simulink model "sampleModel1487"  (R2023a)
settings: Solver=VariableStepAuto  StartTime=0.0  StopTime=10.0  RelTol=1e-3
libraries: hdlsllib x4, simulink x2
settings Model: Creator=user1  LastModifiedBy=user1

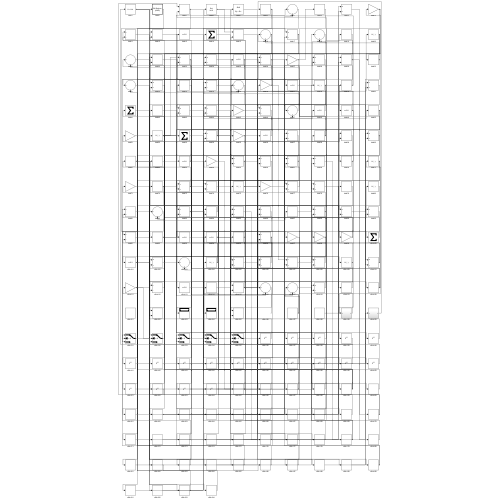
[thumbnail: Simulink's stored preview of the top-level diagram]
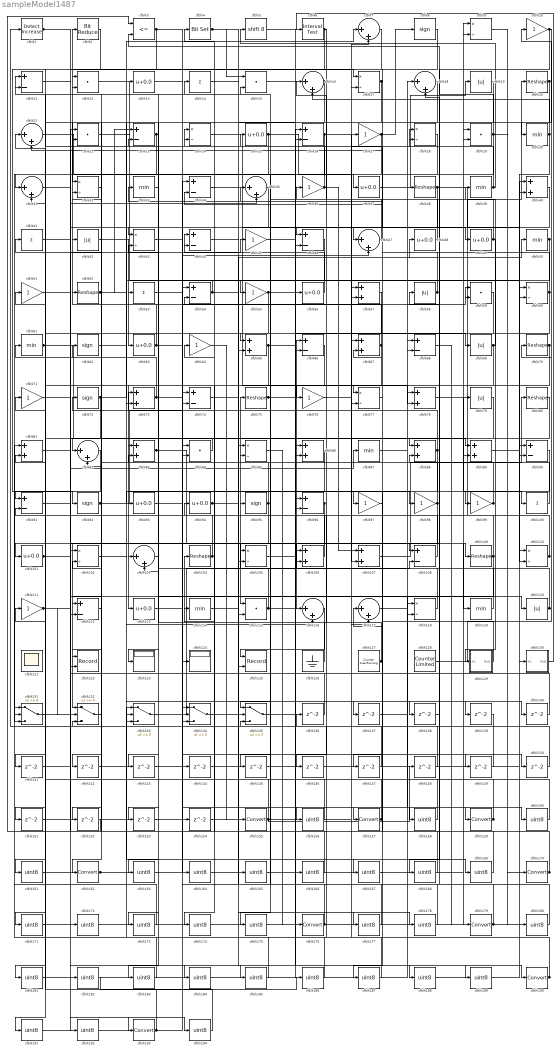
== system sampleModel1487 ==
  cfblk1 : simulink/Logic and Bit Operations/Detect Increase  vinit=0.0  OutDataTypeStr=boolean
      settings: LibrarySourceBlock=|
      | hdlsllib/Logic and Bit
      | Operations/Detect
      | Increase
  cfblk{10,27,36,45,51,55,64,71,76,97..99,111} (13 alike) : Gain
  cfblk{14,41,53,100} (4 alike) : Sum  Inputs=+
  cfblk{13,25,37,48..49,56,63,93..94,101,113} (11 alike) : Bias  Bias=0.0  SaturateOnIntegerOverflow=off
  cfblk{9,17,24,28,32,43,60,77,85,102,105,110,118} (13 alike) : Product  Inputs=*/  RndMeth=Zero  SaturateOnIntegerOverflow=on
  cfblk{7,16,18,21,31,35,47,82,103,116..117} (11 alike) : Sum  Inputs=|++
  cfblk{20,38,52,70,75,80,104,109} (8 alike) : Reshape
  cfblk{40,57,65,67,73,78,81,83,86,88..89,106..107} (13 alike) : Sum
  cfblk{11,23,26,34,44,46,54,66,68,74,90..91,96,108,112} (15 alike) : Sum  Inputs=+-
  cfblk{30,33,39,50,61,87,114,119} (8 alike) : MinMax
  cfblk{12,15,22,29,59,84,115} (7 alike) : DotProduct  OutDataTypeStr=Inherit: Inherit via internal rule
  cfblk{19,42,58,69,79,120} (6 alike) : Abs  SaturateOnIntegerOverflow=off
  cfblk121 : Scope
      settings: Floating=on
  cfblk122 : Record  FileSettingsInternal="{\"entries\":[{\"content\":{\"excelSettings\":{\"content\":{},\"type\":\"Streamout.ExcelSettings\"}},\"type\":\"Streamout.FileSettingStorage\",\"uuid\":\"\"}],\"packageUris\":[\"http:\\/\\/schema.mathworks.com\\/mf0\\/streamout_blocks\\/R2020a\"],\"version\":\"1.0\"}"  Layout=[1 1]  SignalsInternal="{\"entries\":[{\"content\":{\"signals\":[{\"content\":{\"blockPath\":[],\"dimensions\":[1],\"domain\":\"\",\"lineColor\":\"#a2142f\",\"plots\":[1],\"port\":1,\"signalID\":1175,\"signalName\":\"XY Graph:1\"},\"type\":\"RecordBlkView.Signal\",\"uuid\":\"\"},{\"content\":{\"blockPath\":[],\"dimensions\":[1],\"domain\":\"\",\"lineColor\":\"#139fff\",\"plots\":[1],\"port\":2,\"signalID\":1178,\"signalName\":\"XY Graph:2\"},\"type\":\"RecordBlkView.Signal\",\"uuid\":\"\"}]},\"type\":\"RecordBlkView.InputSignals\",\"uuid\":\"\"}],\"packageUris\":[\"http:\\/\\/schema.mathworks.com\\/mf0\\/streamout_blocks\\/R2020a\"],\"version\":\"1.0\"}"  VisualizationBindings="{\"xyplotplugin\":{\"info\":[{\"series\":[{\"bindingParametersList\":[{\"parameter\":\"X-Axis\",\"signalID\":1175,\"signalName\":\"XY Graph:1\"},{\"parameter\":\"Y-Axis\",\"signalID\":1178,\"signalName\":\"XY Graph:2\"}],\"seriesID\":46251}],\"subplotID\":1}]}}"  CompatibilityTag=XY  st=-1
  cfblk123 : Display
  cfblk124 : Display
  cfblk125 : Record  FileSettingsInternal="{\"entries\":[{\"content\":{\"excelSettings\":{\"content\":{},\"type\":\"Streamout.ExcelSettings\"}},\"type\":\"Streamout.FileSettingStorage\",\"uuid\":\"\"}],\"packageUris\":[\"http:\\/\\/schema.mathworks.com\\/mf0\\/streamout_blocks\\/R2020a\"],\"version\":\"1.0\"}"  Layout=[1 1]  SignalsInternal="{\"entries\":[{\"content\":{\"signals\":[{\"content\":{\"blockPath\":[],\"dimensions\":[1],\"domain\":\"\",\"lineColor\":\"#a2142f\",\"plots\":[1],\"port\":1,\"signalID\":1183,\"signalName\":\"XY Graph:1\"},\"type\":\"RecordBlkView.Signal\",\"uuid\":\"\"},{\"content\":{\"blockPath\":[],\"dimensions\":[1],\"domain\":\"\",\"lineColor\":\"#139fff\",\"plots\":[1],\"port\":2,\"signalID\":1186,\"signalName\":\"XY Graph:2\"},\"type\":\"RecordBlkView.Signal\",\"uuid\":\"\"}]},\"type\":\"RecordBlkView.InputSignals\",\"uuid\":\"\"}],\"packageUris\":[\"http:\\/\\/schema.mathworks.com\\/mf0\\/streamout_blocks\\/R2020a\"],\"version\":\"1.0\"}"  VisualizationBindings="{\"xyplotplugin\":{\"info\":[{\"series\":[{\"bindingParametersList\":[{\"parameter\":\"X-Axis\",\"signalID\":1183,\"signalName\":\"XY Graph:1\"},{\"parameter\":\"Y-Axis\",\"signalID\":1186,\"signalName\":\"XY Graph:2\"}],\"seriesID\":58959}],\"subplotID\":1}]}}"  CompatibilityTag=XY  st=-1
  cfblk126 : Ground
  cfblk127 : hdlsllib/Sources/Counter Free-Running  NumBits=16  tsamp=-1
  cfblk128 : hdlsllib/Sources/Counter Limited  uplimit=7  tsamp=-1
  cfblk129 : Subsystem
      settings: LibrarySourceBlock=|
      | hdlsllib/Ports &
      | Subsystems/Subsystem
  cfblk130 : Subsystem
      settings: LibrarySourceBlock=|
      | hdlsllib/Ports &
      | Subsystems/Subsystem
  cfblk{131..135} (5 alike) : Switch  SaturateOnIntegerOverflow=off  InputSameDT=off
  cfblk{136..154} (19 alike) : Delay  SampleTime=1
  cfblk{155,157,159,162,170,176,179,190,193} (9 alike) : DataTypeConversion  SaturateOnIntegerOverflow=off  RndMeth=Floor
  cfblk{156,158,160..161,163..169,171..175,177..178,180..189,191..192,194} (31 alike) : DataTypeConversion  OutDataTypeStr=uint8  SaturateOnIntegerOverflow=off  RndMeth=Floor
  cfblk2 : hdlsllib/Logic and Bit Operations/Bit Reduce  mode=AND
  cfblk3 : RelationalOperator  Operator=<=  OutDataTypeStr=boolean  InputSameDT=off
  cfblk4 : simulink/Logic and Bit Operations/Bit Set  iBit=0
      settings: LibrarySourceBlock=|
      | hdlsllib/Logic and Bit
      | Operations/Bit Set
  cfblk5 : ArithShift  BitShiftNumber=8
  cfblk6 : hdlsllib/Logic and Bit Operations/Interval Test  IntervalClosedRight=on  uplimit=0.5  IntervalClosedLeft=on  lowlimit=-0.5  OutDataTypeStr=boolean
  cfblk{8,62,72,92,95} (5 alike) : Signum
  wires:
  cfblk47/1 -> cfblk11/1
  cfblk77/1 -> cfblk37/1
  cfblk37/1 -> cfblk19/1
  cfblk2/1 -> cfblk92/1
  cfblk4/1 -> cfblk15/1, cfblk26/2
  cfblk39/1 -> cfblk5/1, cfblk28/2
  cfblk104/1 -> cfblk41/1, cfblk94/1
  cfblk109/1 -> cfblk20/1, cfblk153/1
  cfblk67/1 -> cfblk2/1, cfblk93/1
  cfblk55/1 -> cfblk91/1, cfblk69/1
  cfblk126/1 -> cfblk104/1
  cfblk84/1 -> cfblk82/1
  cfblk74/1 -> cfblk190/1
  cfblk48/1 -> cfblk36/1
  cfblk65/1 -> cfblk113/1, cfblk59/1
  cfblk89/1 -> cfblk40/1
  cfblk119/1 -> cfblk75/1
  cfblk118/1 -> cfblk66/1
  cfblk128/1 -> cfblk10/1
  cfblk34/1 -> cfblk77/1
  cfblk17/1 -> cfblk32/1, cfblk46/1
  cfblk36/1 -> cfblk11/2, cfblk107/1
  cfblk8/1 -> cfblk47/1
  cfblk95/1 -> cfblk132/1, cfblk62/1
  cfblk32/1 -> cfblk122/1
  cfblk96/1 -> cfblk116/1, cfblk161/1
  cfblk127/1 -> cfblk73/1, cfblk91/2
  cfblk50/1 -> cfblk65/2, cfblk183/1
  cfblk9/1 -> cfblk170/1
  cfblk130/1(Out1) -> cfblk6/1
  cfblk120/1 -> cfblk12/1, cfblk70/1, cfblk43/2
  cfblk26/1 -> cfblk123/1, cfblk78/2
  cfblk16/1 -> cfblk43/1, cfblk191/1
  cfblk73/1 -> cfblk21/1, cfblk98/1
  cfblk21/1 -> cfblk66/2
  cfblk12/1 -> cfblk60/2
  cfblk112/1 -> cfblk32/2
  cfblk24/1 -> cfblk49/1
  cfblk116/1 -> cfblk125/1
  cfblk61/1 -> cfblk88/1, cfblk118/2
  cfblk29/1 -> cfblk31/1, cfblk3/2, cfblk180/1
  cfblk133/1 -> cfblk27/1
  cfblk20/1 -> cfblk133/3, cfblk152/1, cfblk168/1
  cfblk54/1 -> cfblk53/1, cfblk89/1, cfblk138/1
  cfblk106/1 -> cfblk44/1
  cfblk38/1 -> cfblk110/1, cfblk65/1, cfblk146/1
  cfblk72/1 -> cfblk13/1, cfblk181/1
  cfblk27/1 -> cfblk8/1, cfblk175/1
  cfblk107/1 -> cfblk80/1
  cfblk5/1 -> cfblk109/1
  cfblk111/1 -> cfblk132/2, cfblk194/1
  cfblk132/1 -> cfblk72/1
  cfblk98/1 -> cfblk115/1, cfblk83/2, cfblk96/2
  cfblk33/1 -> cfblk103/1
  cfblk18/1 -> cfblk82/2
  cfblk25/1 -> cfblk77/2, cfblk141/1, cfblk142/1
  cfblk129/1(Out1) -> cfblk21/2
  cfblk58/1 -> cfblk25/1, cfblk34/2
  cfblk83/1 -> cfblk119/1, cfblk59/2
  cfblk108/1 -> cfblk24/1
  cfblk101/1 -> cfblk45/1, cfblk189/1
  cfblk10/1 -> cfblk108/1, cfblk30/1
  cfblk42/1 -> cfblk63/1
  cfblk79/1 -> cfblk135/1
  cfblk68/1 -> cfblk179/1
  cfblk60/1 -> cfblk33/1, cfblk103/2, cfblk107/2
  cfblk57/1 -> cfblk162/1
  cfblk64/1 -> cfblk155/1
  cfblk78/1 -> cfblk100/1
  cfblk46/1 -> cfblk73/2
  cfblk100/1 -> cfblk61/1
  cfblk22/1 -> cfblk96/1
  cfblk76/1 -> cfblk28/1
  cfblk28/1 -> cfblk125/2
  cfblk56/1 -> cfblk4/1
  cfblk75/1 -> cfblk48/1, cfblk140/1
  cfblk99/1 -> cfblk35/1, cfblk24/2
  cfblk44/1 -> cfblk120/1
  cfblk94/1 -> cfblk50/1, cfblk177/1
  cfblk30/1 -> cfblk110/2, cfblk16/2
  cfblk19/1 -> cfblk122/2
  cfblk62/1 -> cfblk116/2
  cfblk117/1 -> cfblk159/1
  cfblk131/1 -> cfblk35/2
  cfblk87/1 -> cfblk18/1
  cfblk85/1 -> cfblk176/1
  cfblk91/1 -> cfblk87/1
  cfblk23/1 -> cfblk131/3, cfblk143/1
  cfblk69/1 -> cfblk39/1, cfblk84/2
  cfblk63/1 -> cfblk52/1, cfblk149/1
  cfblk11/1 -> cfblk105/1
  cfblk82/1 -> cfblk131/2
  cfblk80/1 -> cfblk112/1
  cfblk52/1 -> cfblk7/1, cfblk23/1, cfblk135/2, cfblk137/1
  cfblk49/1 -> cfblk129/1(In1), cfblk16/1
  cfblk110/1 -> cfblk95/1, cfblk23/2
  cfblk43/1 -> cfblk47/2
  cfblk13/1 -> cfblk124/1
  cfblk6/1 -> cfblk76/1, cfblk134/2
  cfblk35/1 -> cfblk112/2
  cfblk92/1 -> cfblk54/1, cfblk97/1
  cfblk14/1 -> cfblk157/1
  cfblk1/1 -> cfblk17/1, cfblk106/2, cfblk89/2
  cfblk40/1 -> cfblk83/1
  cfblk115/1 -> cfblk106/1, cfblk54/2, cfblk108/2, cfblk178/1
  cfblk3/1 -> cfblk55/1, cfblk151/1
  cfblk71/1 -> cfblk193/1
  cfblk88/1 -> cfblk22/2, cfblk134/3
  cfblk70/1 -> cfblk101/1, cfblk99/1
  cfblk136/1 -> cfblk15/2
  cfblk138/1 -> cfblk88/2
  cfblk53/1 -> cfblk139/1
  cfblk139/1 -> cfblk1/1
  cfblk140/1 -> cfblk22/1
  cfblk142/1 -> cfblk7/2
  cfblk113/1 -> cfblk144/1
  cfblk144/1 -> cfblk105/2
  cfblk59/1 -> cfblk145/1
  cfblk145/1 -> cfblk60/1
  cfblk146/1 -> cfblk40/2
  cfblk97/1 -> cfblk147/1
  cfblk147/1 -> cfblk44/2
  cfblk148/1 -> cfblk26/1
  cfblk149/1 -> cfblk78/1
  cfblk134/1 -> cfblk150/1
  cfblk150/1 -> cfblk12/2
  cfblk151/1 -> cfblk17/2
  cfblk152/1 -> cfblk3/1
  cfblk153/1 -> cfblk46/2
  cfblk154/1 -> cfblk115/2
  cfblk155/1 -> cfblk148/1, cfblk84/1
  cfblk93/1 -> cfblk156/1
  cfblk156/1 -> cfblk64/1
  cfblk157/1 -> cfblk132/3, cfblk111/1
  cfblk45/1 -> cfblk158/1
  cfblk158/1 -> cfblk14/1
  cfblk159/1 -> cfblk133/2, cfblk18/2, cfblk34/1, cfblk42/1
  cfblk137/1 -> cfblk160/1
  cfblk160/1 -> cfblk117/1
  cfblk161/1 -> cfblk117/2
  cfblk162/1 -> cfblk29/2, cfblk29/1
  cfblk103/1 -> cfblk163/1
  cfblk163/1 -> cfblk57/1
  cfblk143/1 -> cfblk164/1
  cfblk164/1 -> cfblk57/2
  cfblk114/1 -> cfblk165/1
  cfblk165/1 -> cfblk38/1
  cfblk105/1 -> cfblk166/1
  cfblk166/1 -> cfblk114/1
  cfblk102/1 -> cfblk167/1
  cfblk167/1 -> cfblk79/1
  cfblk168/1 -> cfblk102/1
  cfblk15/1 -> cfblk169/1
  cfblk169/1 -> cfblk102/2
  cfblk170/1 -> cfblk135/3, cfblk67/2
  cfblk7/1 -> cfblk171/1
  cfblk171/1 -> cfblk9/1
  cfblk141/1 -> cfblk172/1
  cfblk172/1 -> cfblk9/2
  cfblk86/1 -> cfblk173/1
  cfblk173/1 -> cfblk131/1
  cfblk66/1 -> cfblk174/1
  cfblk174/1 -> cfblk86/1
  cfblk175/1 -> cfblk86/2
  cfblk176/1 -> cfblk134/1, cfblk130/1(In1)
  cfblk177/1 -> cfblk85/1
  cfblk178/1 -> cfblk85/2
  cfblk179/1 -> cfblk118/1, cfblk58/1
  cfblk180/1 -> cfblk68/1
  cfblk181/1 -> cfblk68/2
  cfblk51/1 -> cfblk182/1
  cfblk183/1 -> cfblk51/1
  cfblk81/1 -> cfblk184/1
  cfblk184/1 -> cfblk56/1
  cfblk31/1 -> cfblk185/1
  cfblk185/1 -> cfblk81/1
  cfblk182/1 -> cfblk186/1
  cfblk186/1 -> cfblk81/2
  cfblk90/1 -> cfblk187/1
  cfblk187/1 -> cfblk136/1
  cfblk135/1 -> cfblk188/1
  cfblk188/1 -> cfblk90/1
  cfblk189/1 -> cfblk90/2
  cfblk190/1 -> cfblk133/1, cfblk67/1
  cfblk191/1 -> cfblk74/1
  cfblk41/1 -> cfblk192/1
  cfblk192/1 -> cfblk74/2
  cfblk193/1 -> cfblk154/1, cfblk31/2
  cfblk194/1 -> cfblk71/1

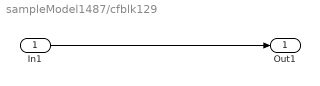
== system sampleModel1487/cfblk129 ==
  In1 : Inport
  Out1 : Outport
  wires:
  In1/1 -> Out1/1

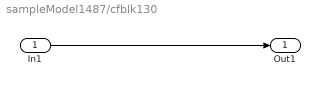
== system sampleModel1487/cfblk130 ==
  In1 : Inport
  Out1 : Outport
  wires:
  In1/1 -> Out1/1
